simulink model "rocketManipulator"  (R2020b)
settings: Solver=VariableStepAuto  StartTime=0.0  StopTime=inf  RelTol=1e-3
libraries: vrlib x3
settings Model: Creator=bean657  LastModifiedBy=Andreas

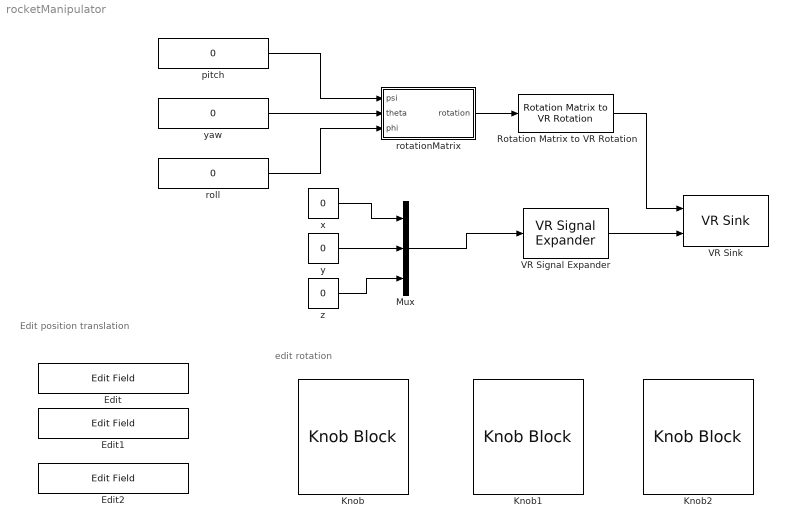
== system rocketManipulator ==
  note: edit rotation
  note: Edit position translation
  Edit : EditField  LabelPosition=Hide  ShowInitialText=on  Alignment=Center
  Edit1 : EditField  LabelPosition=Hide  ShowInitialText=on  Alignment=Center
  Edit2 : EditField  LabelPosition=Hide  ShowInitialText=on  Alignment=Center
  Knob : KnobBlock  ScaleMin=-1.57  ScaleMax=1.57  TickInterval=0.55
  Knob1 : KnobBlock  ScaleMin=-1.57  ScaleMax=1.57  TickInterval=0.55
  Knob2 : KnobBlock  ScaleMin=-1.57  ScaleMax=1.57  TickInterval=0.55
  Mux : Mux  Inputs=3
  Rotation Matrix to VR Rotation : vrlib/Utilities/Rotation Matrix to VR Rotation  maxzero=1e-12
      settings: SourceProductBaseCode=SL
  VR Signal Expander : vrlib/VR Signal Expander  outwidth=3  outidx=[1 2 3]
  VR Sink : vrlib/VR Sink  InstantiateOnLoad=on  SampleTime=0.1  ViewEnable=on  RemoteChange=off  RemoteView=off  FieldsWritten=Shuttle.rotation.4.1.1.double#Shuttle.translation.3.1.1.double  WorldFileName=rocketWorld.x3d  AutoView=off  VideoDimensions=[]  AllowVariableSize=off
  pitch : Constant  Value=0
  roll : Constant  Value=0
  rotationMatrix : MATLAB Function  TreatAsAtomicUnit=on
  x : Constant  Value=0
  y : Constant  Value=0
  yaw : Constant  Value=0
  z : Constant  Value=0
  wires:
  VR Signal Expander/1 -> VR Sink/2
  rotationMatrix/1(rotation) -> Rotation Matrix to VR Rotation/1
  pitch/1 -> rotationMatrix/1(psi)
  yaw/1 -> rotationMatrix/2(theta)
  roll/1 -> rotationMatrix/3(phi)
  Rotation Matrix to VR Rotation/1 -> VR Sink/1
  Mux/1 -> VR Signal Expander/1
  x/1 -> Mux/1
  y/1 -> Mux/2
  z/1 -> Mux/3

== matlab function rocketManipulator/rotationMatrix ==
  data: psi input; rotation output; theta input; phi input
function rotation = fcn(psi,theta,phi)%yaw pitch roll

%yaw matrix
R3   = [ cos(psi) sin(psi) 0; 
             -sin(psi) cos(psi) 0; 
             0 0 1];
%pitch matrix
R2   = [cos(theta) 0 -sin(theta); 
        0  1           0; 
        sin(theta) 0  cos(theta)];
%roll matrix         
R1    = [1        0          0; 
         0  cos(phi)  sin(phi);
         0 -sin(phi)  cos(phi)];
         
         rotation = R1 * R2 * R3;
end
